simulink model "Tracker_with_Position_Control_Sine_ESP32"  (R2024b)
settings: Solver=FixedStepDiscrete  StartTime=0.0  StopTime=inf  FixedStep=0.005  RelTol=1e-3  EnableMultiTasking=on
libraries: arduinolib x6, simulink x2, arduinosensorlib x2, simulink_extras x2, slpidlib x2
settings Model: ExtModeTrigDuration=2  Creator=yoany  LastModifiedBy=shaha
settings SolverCC: AutoInsertRateTranBlk=on
settings OptimizationCC: DefaultUnderspecifiedDataType=single  EnhancedBackFolding=on  PassReuseOutputArgsThreshold=0  MaxStackSize=64  OptimizeBlockOrder=speed  DifferentSizesBufferReuse=on
settings DebuggingCC: MultiTaskRateTransMsg=warning  ParameterPrecisionLossMsg=none  ParameterTunabilityLossMsg=error
settings HardwareCC: ProdBitPerPointer=32  ProdBitPerSizeT=32  ProdBitPerPtrDiffT=32  ProdLargestAtomicInteger=Long  ProdLargestAtomicFloat=Double  ProdWordSize=32  ProdHWDeviceType=ARM Compatible->ARM Cortex
settings SFSimCC: MATLABDynamicMemAlloc=off
settings RTWCC: Description=Embedded Coder  SystemTargetFile=ert.tlc  HardwareBoard=ESP32-WROOM(Arduino Compatible)  TLCOptions="-aInlineSetEventsForThisBaseRateFcn=TLC_FALSE -aSuppressMultiTaskScheduler=TLC_FALSE    -aRateBasedStepFcn=0"  TemplateMakefile=ert_default_tmf  Toolchain=ESP32  BuildConfiguration=Faster Runs  GPUComputeCapability=3.5
settings CodeAppCC: ForceParamTrailComments=on  OperatorAnnotations=on
settings ERTTargetCC: ERTCustomFileBanners=off  SupportContinuousTime=on  SupportNonInlinedSFcns=on  RemoveResetFunc=off  SupportVariableSizeSignals=on  ModelStepFunctionPrototypeControlCompliant=off  ExtModeTransport=3  ExtModeStaticAlloc=on  ExtModeAutomaticAllocSize=off  ExtModeStaticAllocSize=65536  ExtModeMexFile=ext_xcp  ExtModeIntrfLevel=Level2 - Open  InlinedParameterPlacement=Hierarchical  DynamicArrayContainerType=coder::array

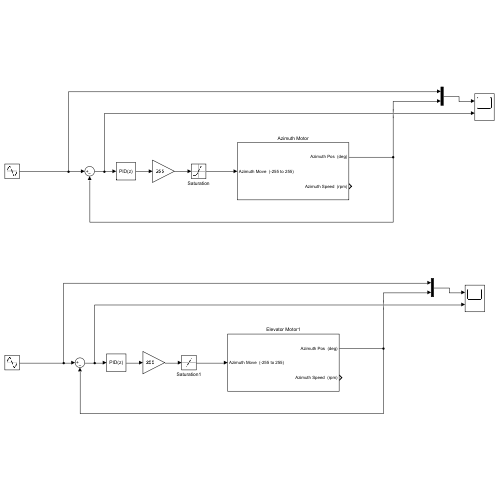
[thumbnail: Simulink's stored preview of the top-level diagram]
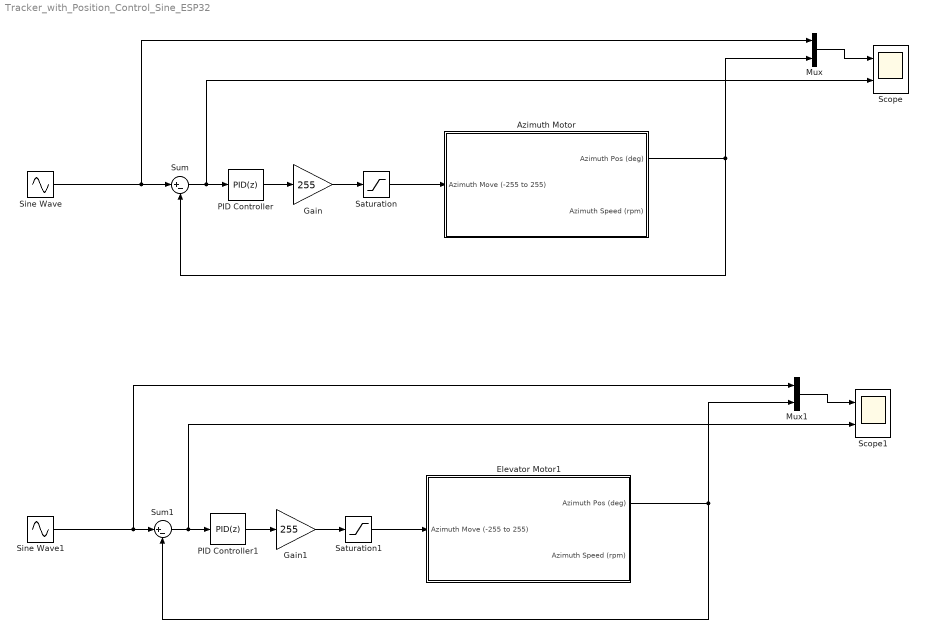
== system Tracker_with_Position_Control_Sine_ESP32 ==
  Azimuth Motor : Subsystem
  Elevator Motor1 : Subsystem
  Gain : Gain  Gain=255
  Gain1 : Gain  Gain=255
  Mux : Mux  Inputs=2
  Mux1 : Mux  Inputs=2
  PID Controller : slpidlib/PID Controller  Controller=PID  Form=Parallel  TimeDomain=Discrete-time  UseExternalTs=off  SampleTime=0.01  IntegratorMethod=Forward Euler  FilterMethod=Forward Euler  ControllerParametersSource=internal  P=0.01  I=0.005  UseKiTs=off  D=0  UseExternalDerivativeSource=off  N=0  UseFilter=on  TunerSelectOption=Transfer Function Based (PID Tuner App)  InitialConditionSource=internal  InitialConditionForIntegrator=0  InitialConditionForFilter=0  DifferentiatorICPrevScaledInput=0  ExternalReset=none  TrackingMode=off  Kt=1  LimitOutput=off  SatLimitsSource=internal  UpperSaturationLimit=255  LowerSaturationLimit=-255  LinearizeAsGain=on  AntiWindupMode=none  Kb=1  LimitIntegrator=off  UpperIntegratorSaturationLimit=inf  LowerIntegratorSaturationLimit=-inf  POutMin=[]  POutMax=[]  IOutMin=[]  IOutMax=[]  DOutMin=[]  DOutMax=[]  NOutMin=[]  NOutMax=[]  SumOutMin=[]  SumOutMax=[]  SaturationOutMin=[]  SaturationOutMax=[]  PParamMin=[]  PParamMax=[]  IParamMin=[]  IParamMax=[]  DParamMin=[]  DParamMax=[]  NParamMin=[]  NParamMax=[]  KbParamMin=[]  KbParamMax=[]  KtParamMin=[]  KtParamMax=[]  KbOutMin=[]  KbOutMax=[]  KtOutMin=[]  KtOutMax=[]  IntegratorOutMin=[]  IntegratorOutMax=[]  FilterOutMin=[]  FilterOutMax=[]  SumI1OutMin=[]  SumI1OutMax=[]  SumI2OutMin=[]  SumI2OutMax=[]  SumI3OutMin=[]  SumI3OutMax=[]  SumI4OutMin=[]  SumI4OutMax=[]  SumDOutMin=[]  SumDOutMax=[]  DifferentiatorOutMin=[]  DifferentiatorOutMax=[]  FilterDiffOutCoefMin=[]  FilterDiffOutCoefMax=[]  ReciprocalOutMin=[]  ReciprocalOutMax=[]  SumDenOutMin=[]  SumDenOutMax=[]  SumNumOutMin=[]  SumNumOutMax=[]  DivideOutMin=[]  DivideOutMax=[]  UdiffTsProdOutMin=[]  UdiffTsProdOutMax=[]  NTsProdOutMin=[]  NTsProdOutMax=[]  UintegralTsProdOutMin=[]  UintegralTsProdOutMax=[]  UngainTsProdOutMin=[]  UngainTsProdOutMax=[]  ClampingZeroOutDataTypeStr=Inherit: Inherit via back propagation  ClampingZeroOutMin=[]  ClampingZeroOutMax=[]  FilterDenConstantOutDataTypeStr=Inherit: Inherit via back propagation  FilterDenConstantOutMin=[]  FilterDenConstantOutMax=[]  PCopyOutDataTypeStr=Inherit: Inherit via back propagation  PCopyOutMin=[]  PCopyOutMax=[]  NCopyOutDataTypeStr=Inherit: Inherit via back propagation  NCopyOutMin=[]  NCopyOutMax=[]  IntegratorContinuousStateAttributes=''  IntegratorStateMustResolveToSignalObject=off  IntegratorRTWStateStorageClass=Auto  FilterContinuousStateAttributes=''  FilterStateMustResolveToSignalObject=off  FilterRTWStateStorageClass=Auto  ParallelPVariant=InternalParameters  IdealPVariant=Disabled  IVariant=InternalParameters  DVariant=InternalParameters  IntegratorVariant=Discrete  SatVariant=Disabled  AWVariant=Passthrough  PCopyVariant=Disabled  TRVariant=Disabled  FdbkBlocksVariant=Forward  IdealPFdbkVariant=Disabled  SatFdbkVariant=Disabled  DerivativeFilterVariant=ForwardEulerFilter  NVariant=InternalParameters  NCopyVariant=Disabled  FilterICVariant=InternalICsFilter  IntegratorICVariant=InternalICs  ExternalResetVariant=Disabled  TRSumVariant=Passthrough  SumFdbkVariant=Disabled  SumVariant=Sum_PID  TsampFilterVariant=InternalTs  TsampNgainVariant=Passthrough  TsampIntegralVariant=Disabled_SignalSpec  ExternalSaturationOutDataTypeStr=Inherit: Same as second input  DerivativeSourceVariant=ErrorSignal  PreIntVariant=InternalPreInt
  PID Controller1 : slpidlib/PID Controller  Controller=PID  Form=Parallel  TimeDomain=Discrete-time  UseExternalTs=off  SampleTime=0.01  IntegratorMethod=Forward Euler  FilterMethod=Forward Euler  ControllerParametersSource=internal  P=0.01  I=0.005  UseKiTs=off  D=0  UseExternalDerivativeSource=off  N=0  UseFilter=on  TunerSelectOption=Transfer Function Based (PID Tuner App)  InitialConditionSource=internal  InitialConditionForIntegrator=0  InitialConditionForFilter=0  DifferentiatorICPrevScaledInput=0  ExternalReset=none  TrackingMode=off  Kt=1  LimitOutput=off  SatLimitsSource=internal  UpperSaturationLimit=255  LowerSaturationLimit=-255  LinearizeAsGain=on  AntiWindupMode=none  Kb=1  LimitIntegrator=off  UpperIntegratorSaturationLimit=inf  LowerIntegratorSaturationLimit=-inf  POutMin=[]  POutMax=[]  IOutMin=[]  IOutMax=[]  DOutMin=[]  DOutMax=[]  NOutMin=[]  NOutMax=[]  SumOutMin=[]  SumOutMax=[]  SaturationOutMin=[]  SaturationOutMax=[]  PParamMin=[]  PParamMax=[]  IParamMin=[]  IParamMax=[]  DParamMin=[]  DParamMax=[]  NParamMin=[]  NParamMax=[]  KbParamMin=[]  KbParamMax=[]  KtParamMin=[]  KtParamMax=[]  KbOutMin=[]  KbOutMax=[]  KtOutMin=[]  KtOutMax=[]  IntegratorOutMin=[]  IntegratorOutMax=[]  FilterOutMin=[]  FilterOutMax=[]  SumI1OutMin=[]  SumI1OutMax=[]  SumI2OutMin=[]  SumI2OutMax=[]  SumI3OutMin=[]  SumI3OutMax=[]  SumI4OutMin=[]  SumI4OutMax=[]  SumDOutMin=[]  SumDOutMax=[]  DifferentiatorOutMin=[]  DifferentiatorOutMax=[]  FilterDiffOutCoefMin=[]  FilterDiffOutCoefMax=[]  ReciprocalOutMin=[]  ReciprocalOutMax=[]  SumDenOutMin=[]  SumDenOutMax=[]  SumNumOutMin=[]  SumNumOutMax=[]  DivideOutMin=[]  DivideOutMax=[]  UdiffTsProdOutMin=[]  UdiffTsProdOutMax=[]  NTsProdOutMin=[]  NTsProdOutMax=[]  UintegralTsProdOutMin=[]  UintegralTsProdOutMax=[]  UngainTsProdOutMin=[]  UngainTsProdOutMax=[]  ClampingZeroOutDataTypeStr=Inherit: Inherit via back propagation  ClampingZeroOutMin=[]  ClampingZeroOutMax=[]  FilterDenConstantOutDataTypeStr=Inherit: Inherit via back propagation  FilterDenConstantOutMin=[]  FilterDenConstantOutMax=[]  PCopyOutDataTypeStr=Inherit: Inherit via back propagation  PCopyOutMin=[]  PCopyOutMax=[]  NCopyOutDataTypeStr=Inherit: Inherit via back propagation  NCopyOutMin=[]  NCopyOutMax=[]  IntegratorContinuousStateAttributes=''  IntegratorStateMustResolveToSignalObject=off  IntegratorRTWStateStorageClass=Auto  FilterContinuousStateAttributes=''  FilterStateMustResolveToSignalObject=off  FilterRTWStateStorageClass=Auto  ParallelPVariant=InternalParameters  IdealPVariant=Disabled  IVariant=InternalParameters  DVariant=InternalParameters  IntegratorVariant=Discrete  SatVariant=Disabled  AWVariant=Passthrough  PCopyVariant=Disabled  TRVariant=Disabled  FdbkBlocksVariant=Forward  IdealPFdbkVariant=Disabled  SatFdbkVariant=Disabled  DerivativeFilterVariant=ForwardEulerFilter  NVariant=InternalParameters  NCopyVariant=Disabled  FilterICVariant=InternalICsFilter  IntegratorICVariant=InternalICs  ExternalResetVariant=Disabled  TRSumVariant=Passthrough  SumFdbkVariant=Disabled  SumVariant=Sum_PID  TsampFilterVariant=InternalTs  TsampNgainVariant=Passthrough  TsampIntegralVariant=Disabled_SignalSpec  ExternalSaturationOutDataTypeStr=Inherit: Same as second input  DerivativeSourceVariant=ErrorSignal  PreIntVariant=InternalPreInt
  Saturation : Saturate  UpperLimit=255  LowerLimit=-255
  Saturation1 : Saturate  UpperLimit=255  LowerLimit=-255
  Scope : Scope  NumInputPorts=2
  Scope1 : Scope  NumInputPorts=2
  Sine Wave : Sin  Amplitude=90  Frequency=pi/2  SampleTime=0
  Sine Wave1 : Sin  Amplitude=0  Frequency=pi/2  SampleTime=0
  Sum : Sum  Inputs=|+-
  Sum1 : Sum  Inputs=|+-
  wires:
  Sum/1 -> Scope/2, PID Controller/1
  Azimuth Motor/1(Azimuth Pos (deg)) -> Sum/2, Mux/2
  Saturation/1 -> Azimuth Motor/1(Azimuth Move (-255 to 255))
  Gain/1 -> Saturation/1
  PID Controller/1 -> Gain/1
  Mux/1 -> Scope/1
  Mux1/1 -> Scope1/1
  PID Controller1/1 -> Gain1/1
  Elevator Motor1/1(Azimuth Pos (deg)) -> Sum1/2, Mux1/2
  Gain1/1 -> Saturation1/1
  Sum1/1 -> Scope1/2, PID Controller1/1
  Saturation1/1 -> Elevator Motor1/1(Azimuth Move (-255 to 255))
  Sine Wave/1 -> Mux/1, Sum/1
  Sine Wave1/1 -> Mux1/1, Sum1/1

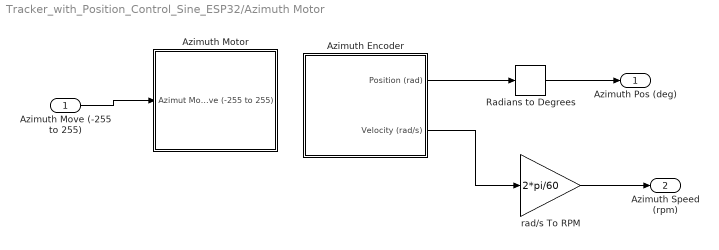
== system Tracker_with_Position_Control_Sine_ESP32/Azimuth Motor ==
  Azimuth Move (-255 to 255) : Inport
  Azimuth Encoder : Subsystem
  Azimuth Motor : Subsystem
  Radians to Degrees : simulink_extras/Transformations/Radians to Degrees
  rad/s To RPM : Gain  Gain=2*pi/60
  Azimuth Pos (deg) : Outport
  Azimuth Speed (rpm) : Outport  Port=2
  wires:
  Azimuth Encoder/2(Velocity (rad/s)) -> rad/s To RPM/1
  Azimuth Encoder/1(Position (rad)) -> Radians to Degrees/1
  Azimuth Move (-255 to 255)/1 -> Azimuth Motor/1(Azimut Move (-255 to 255))
  Radians to Degrees/1 -> Azimuth Pos (deg)/1
  rad/s To RPM/1 -> Azimuth Speed (rpm)/1

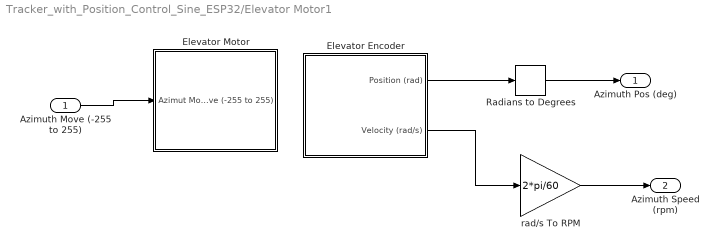
== system Tracker_with_Position_Control_Sine_ESP32/Elevator Motor1 ==
  Azimuth Move (-255 to 255) : Inport
  Elevator Encoder : Subsystem
  Elevator Motor : Subsystem
  Radians to Degrees : simulink_extras/Transformations/Radians to Degrees
  rad/s To RPM : Gain  Gain=2*pi/60
  Azimuth Pos (deg) : Outport
  Azimuth Speed (rpm) : Outport  Port=2
  wires:
  Elevator Encoder/2(Velocity (rad/s)) -> rad/s To RPM/1
  Elevator Encoder/1(Position (rad)) -> Radians to Degrees/1
  Azimuth Move (-255 to 255)/1 -> Elevator Motor/1(Azimut Move (-255 to 255))
  Radians to Degrees/1 -> Azimuth Pos (deg)/1
  rad/s To RPM/1 -> Azimuth Speed (rpm)/1

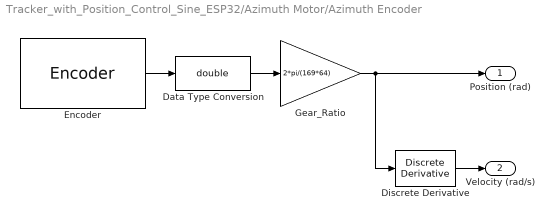
== system Tracker_with_Position_Control_Sine_ESP32/Azimuth Motor/Azimuth Encoder ==
  Data Type Conversion : DataTypeConversion  OutDataTypeStr=double  SaturateOnIntegerOverflow=off  RndMeth=Floor
  Discrete Derivative : simulink/Quick Insert/Discrete/Discrete Derivative  gainval=1.0  ICPrevScaledInput=0.05  OutMin=[]  OutMax=[]  OutDataType=fixdt(1, 16)  OutScaling=2^-10  DoSatur=off
  Encoder : arduinosensorlib/Encoder  InputA=15  InputB=16  Mode=No reset  SampleTime=0.01
  Gear_Ratio : Gain  Gain=2*pi/(169*64)
  Position (rad) : Outport
  Velocity (rad/s) : Outport  Port=2
  wires:
  Gear_Ratio/1 -> Discrete Derivative/1, Position (rad)/1
  Discrete Derivative/1 -> Velocity (rad/s)/1
  Data Type Conversion/1 -> Gear_Ratio/1
  Encoder/1 -> Data Type Conversion/1

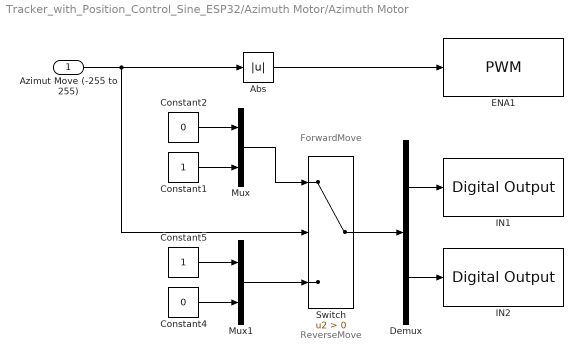
== system Tracker_with_Position_Control_Sine_ESP32/Azimuth Motor/Azimuth Motor ==
  note: ForwardMove
  note: ReverseMove
  Azimut Move (-255 to 255) : Inport
  Abs : Abs  SaturateOnIntegerOverflow=off
  Constant1 : Constant
  Constant2 : Constant  Value=0
  Constant4 : Constant  Value=0
  Constant5 : Constant
  Demux : Demux  Outputs=2
  ENA1 : arduinolib/PWM  pinNumber=18  frequencyType=Default  desiredFrequency=490.2  achievableFrequency=490.2
  IN1 : arduinolib/Digital Output  pinNumber=32  Direction=output  blockPlatform=arduino
  IN2 : arduinolib/Digital Output  pinNumber=33  Direction=output  blockPlatform=arduino
  Mux : Mux  Inputs=2
  Mux1 : Mux  Inputs=2
  Switch : Switch  Criteria=u2 > Threshold  SaturateOnIntegerOverflow=off  InputSameDT=off
  wires:
  Constant5/1 -> Mux1/1
  Mux/1 -> Switch/1
  Azimut Move (-255 to 255)/1 -> Switch/2, Abs/1
  Demux/1 -> IN1/1
  Constant1/1 -> Mux/2
  Constant4/1 -> Mux1/2
  Switch/1 -> Demux/1
  Abs/1 -> ENA1/1
  Demux/2 -> IN2/1
  Mux1/1 -> Switch/3
  Constant2/1 -> Mux/1

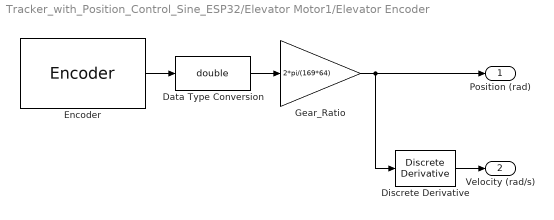
== system Tracker_with_Position_Control_Sine_ESP32/Elevator Motor1/Elevator Encoder ==
  Data Type Conversion : DataTypeConversion  OutDataTypeStr=double  SaturateOnIntegerOverflow=off  RndMeth=Floor
  Discrete Derivative : simulink/Quick Insert/Discrete/Discrete Derivative  gainval=1.0  ICPrevScaledInput=0.05  OutMin=[]  OutMax=[]  OutDataType=fixdt(1, 16)  OutScaling=2^-10  DoSatur=off
  Encoder : arduinosensorlib/Encoder  InputA=5  InputB=4  Mode=No reset  SampleTime=0.01
  Gear_Ratio : Gain  Gain=2*pi/(169*64)
  Position (rad) : Outport
  Velocity (rad/s) : Outport  Port=2
  wires:
  Gear_Ratio/1 -> Discrete Derivative/1, Position (rad)/1
  Discrete Derivative/1 -> Velocity (rad/s)/1
  Data Type Conversion/1 -> Gear_Ratio/1
  Encoder/1 -> Data Type Conversion/1

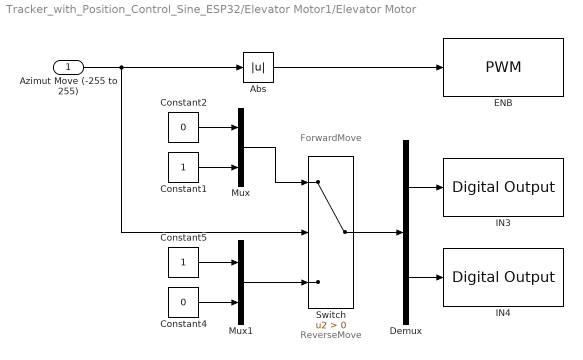
== system Tracker_with_Position_Control_Sine_ESP32/Elevator Motor1/Elevator Motor ==
  note: ForwardMove
  note: ReverseMove
  Azimut Move (-255 to 255) : Inport
  Abs : Abs  SaturateOnIntegerOverflow=off
  Constant1 : Constant
  Constant2 : Constant  Value=0
  Constant4 : Constant  Value=0
  Constant5 : Constant
  Demux : Demux  Outputs=2
  ENB : arduinolib/PWM  pinNumber=26  frequencyType=Default  desiredFrequency=490.2  achievableFrequency=490.2
  IN3 : arduinolib/Digital Output  pinNumber=19  Direction=output  blockPlatform=arduino
  IN4 : arduinolib/Digital Output  pinNumber=25  Direction=output  blockPlatform=arduino
  Mux : Mux  Inputs=2
  Mux1 : Mux  Inputs=2
  Switch : Switch  Criteria=u2 > Threshold  SaturateOnIntegerOverflow=off  InputSameDT=off
  wires:
  Constant5/1 -> Mux1/1
  Mux/1 -> Switch/1
  Azimut Move (-255 to 255)/1 -> Switch/2, Abs/1
  Demux/1 -> IN3/1
  Constant1/1 -> Mux/2
  Constant4/1 -> Mux1/2
  Switch/1 -> Demux/1
  Abs/1 -> ENB/1
  Demux/2 -> IN4/1
  Mux1/1 -> Switch/3
  Constant2/1 -> Mux/1
